simulink library "halout"  (R2021b)
settings: Solver=VariableStepAuto  StartTime=0.0  StopTime=10.0  RelTol=1e-3
undefined symbols (not defined in the file): C_TASK_5MS_S, KHAL_CAN1TxReq_flg, KHAL_CAN2TxReq_flg, KHAL_CAN3TxReq_flg, KHAL_CAN4TxReq_flg, KHAL_CAN5TxReq_flg, KHAL_CAN6TxReq_flg, KHAL_CAN7TxReq_flg, TRUE
libraries: FVT_lib x65, simulink x6
(part 5 of 6)

== system halout/HAL_OUT/CAN2/FD2_CE100_0_0x209/FDCBCMBSDBuzzerCmd ==
  FDCBCMBSDBuzzerCmd : Inport
  Data Type Conversion : DataTypeConversion  OutDataTypeStr=uint8  RndMeth=Round
  CAN2_FDC_BCM_BSD_Buzzer_Cmd : Outport
  wires:
  Data Type Conversion/1 -> CAN2_FDC_BCM_BSD_Buzzer_Cmd/1
  FDCBCMBSDBuzzerCmd/1 -> Data Type Conversion/1

== system halout/HAL_OUT/CAN2/FD2_CE100_0_0x209/FDCBCMBrakeCmd ==
  FDCBCMBrakeCmd : Inport
  Data Type Conversion : DataTypeConversion  OutDataTypeStr=uint8  RndMeth=Round
  CAN2_FDC_BCM_Brake_Cmd : Outport
  wires:
  Data Type Conversion/1 -> CAN2_FDC_BCM_Brake_Cmd/1
  FDCBCMBrakeCmd/1 -> Data Type Conversion/1

== system halout/HAL_OUT/CAN2/FD2_CE100_0_0x209/FDCBCMCallBellCmd ==
  FDCBCMCallBellCmd : Inport
  Data Type Conversion : DataTypeConversion  OutDataTypeStr=uint8  RndMeth=Round
  CAN2_FDC_BCM_CallBell_Cmd : Outport
  wires:
  Data Type Conversion/1 -> CAN2_FDC_BCM_CallBell_Cmd/1
  FDCBCMCallBellCmd/1 -> Data Type Conversion/1

== system halout/HAL_OUT/CAN2/FD2_CE100_0_0x209/FDCBCMDVRSignalLCmd ==
  FDCBCMDVRSignalLCmd : Inport
  Data Type Conversion : DataTypeConversion  OutDataTypeStr=uint8  RndMeth=Round
  CAN2_FDC_BCM_DVRSignalL_Cmd : Outport
  wires:
  Data Type Conversion/1 -> CAN2_FDC_BCM_DVRSignalL_Cmd/1
  FDCBCMDVRSignalLCmd/1 -> Data Type Conversion/1

== system halout/HAL_OUT/CAN2/FD2_CE100_0_0x209/FDCBCMDVRSignalRCmd ==
  FDCBCMDVRSignalRCmd : Inport
  Data Type Conversion : DataTypeConversion  OutDataTypeStr=uint8  RndMeth=Round
  CAN2_FDC_BCM_DVRSignalR_Cmd : Outport
  wires:
  Data Type Conversion/1 -> CAN2_FDC_BCM_DVRSignalR_Cmd/1
  FDCBCMDVRSignalRCmd/1 -> Data Type Conversion/1

== system halout/HAL_OUT/CAN2/FD2_CE100_0_0x209/FDCBCMEmExitSWSta ==
  FDCBCMEmExitSWSta : Inport
  Data Type Conversion : DataTypeConversion  OutDataTypeStr=uint8  RndMeth=Round
  CAN2_FDC_BCM_EmExitSW_Sta : Outport
  wires:
  Data Type Conversion/1 -> CAN2_FDC_BCM_EmExitSW_Sta/1
  FDCBCMEmExitSWSta/1 -> Data Type Conversion/1

== system halout/HAL_OUT/CAN2/FD2_CE100_0_0x209/FDCBCMEmSVCmd ==
  FDCBCMEmSVCmd : Inport
  Data Type Conversion : DataTypeConversion  OutDataTypeStr=uint8  RndMeth=Round
  CAN2_FDC_BCM_EmSV_Cmd : Outport
  wires:
  Data Type Conversion/1 -> CAN2_FDC_BCM_EmSV_Cmd/1
  FDCBCMEmSVCmd/1 -> Data Type Conversion/1

== system halout/HAL_OUT/CAN2/FD2_CE100_0_0x209/FDCBCMFDCloseSVCmd ==
  FDCBCMFDCloseSVCmd : Inport
  Data Type Conversion : DataTypeConversion  OutDataTypeStr=uint8  RndMeth=Round
  CAN2_FDC_BCM_FDCloseSV_Cmd : Outport
  wires:
  Data Type Conversion/1 -> CAN2_FDC_BCM_FDCloseSV_Cmd/1
  FDCBCMFDCloseSVCmd/1 -> Data Type Conversion/1

== system halout/HAL_OUT/CAN2/FD2_CE100_0_0x209/FDCBCMFDOpenSVCmd ==
  FDCBCMFDOpenSVCmd : Inport
  Data Type Conversion : DataTypeConversion  OutDataTypeStr=uint8  RndMeth=Round
  CAN2_FDC_BCM_FDOpenSV_Cmd : Outport
  wires:
  Data Type Conversion/1 -> CAN2_FDC_BCM_FDOpenSV_Cmd/1
  FDCBCMFDOpenSVCmd/1 -> Data Type Conversion/1

== system halout/HAL_OUT/CAN2/FD2_CE100_0_0x209/FDCBCMFDoorSta ==
  FDCBCMFDoorSta : Inport
  Data Type Conversion : DataTypeConversion  OutDataTypeStr=uint8  RndMeth=Round
  CAN2_FDC_BCM_FDoor_Sta : Outport
  wires:
  Data Type Conversion/1 -> CAN2_FDC_BCM_FDoor_Sta/1
  FDCBCMFDoorSta/1 -> Data Type Conversion/1

== system halout/HAL_OUT/CAN2/FD2_CE100_0_0x209/FDCBCMFRoomLpSetSta ==
  FDCBCMFRoomLpSetSta : Inport
  Data Type Conversion : DataTypeConversion  OutDataTypeStr=uint8  RndMeth=Round
  CAN2_FDC_BCM_FRoomLpSet_Sta : Outport
  wires:
  Data Type Conversion/1 -> CAN2_FDC_BCM_FRoomLpSet_Sta/1
  FDCBCMFRoomLpSetSta/1 -> Data Type Conversion/1

== system halout/HAL_OUT/CAN2/FD2_CE100_0_0x209/FDCBCMHBeamCmd ==
  FDCBCMHBeamCmd : Inport
  Data Type Conversion : DataTypeConversion  OutDataTypeStr=uint8  RndMeth=Round
  CAN2_FDC_BCM_HBeam_Cmd : Outport
  wires:
  Data Type Conversion/1 -> CAN2_FDC_BCM_HBeam_Cmd/1
  FDCBCMHBeamCmd/1 -> Data Type Conversion/1

== system halout/HAL_OUT/CAN2/FD2_CE100_0_0x209/FDCBCMHazardSWSta ==
  FDCBCMHazardSWSta : Inport
  Data Type Conversion : DataTypeConversion  OutDataTypeStr=uint8  RndMeth=Round
  CAN2_FDC_BCM_HazardSW_Sta : Outport
  wires:
  Data Type Conversion/1 -> CAN2_FDC_BCM_HazardSW_Sta/1
  FDCBCMHazardSWSta/1 -> Data Type Conversion/1

== system halout/HAL_OUT/CAN2/FD2_CE100_0_0x209/FDCBCMHelpINDCmd ==
  FDCBCMHelpINDCmd : Inport
  Data Type Conversion : DataTypeConversion  OutDataTypeStr=uint8  RndMeth=Round
  CAN2_FDC_BCM_HelpIND_Cmd : Outport
  wires:
  Data Type Conversion/1 -> CAN2_FDC_BCM_HelpIND_Cmd/1
  FDCBCMHelpINDCmd/1 -> Data Type Conversion/1

== system halout/HAL_OUT/CAN2/FD2_CE100_0_0x209/FDCBCMInnerBuzzerCmd ==
  FDCBCMInnerBuzzerCmd : Inport
  Data Type Conversion : DataTypeConversion  OutDataTypeStr=uint8  RndMeth=Round
  CAN2_FDC_BCM_InnerBuzzer_Cmd : Outport
  wires:
  Data Type Conversion/1 -> CAN2_FDC_BCM_InnerBuzzer_Cmd/1
  FDCBCMInnerBuzzerCmd/1 -> Data Type Conversion/1

== system halout/HAL_OUT/CAN2/FD2_CE100_0_0x209/FDCBCMInnerBuzzerModeSta ==
  FDCBCMInnerBuzzerModeSta : Inport
  Data Type Conversion : DataTypeConversion  OutDataTypeStr=uint8  RndMeth=Round
  CAN2_FDC_BCM_InnerBuzzerMode_Sta : Outport
  wires:
  Data Type Conversion/1 -> CAN2_FDC_BCM_InnerBuzzerMode_Sta/1
  FDCBCMInnerBuzzerModeSta/1 -> Data Type Conversion/1

== system halout/HAL_OUT/CAN2/FD2_CE100_0_0x209/FDCBCMInnerCallBellCmd ==
  FDCBCMInnerCallBellCmd : Inport
  Data Type Conversion : DataTypeConversion  OutDataTypeStr=uint8  RndMeth=Round
  CAN2_FDC_BCM_InnerCallBell_Cmd : Outport
  wires:
  Data Type Conversion/1 -> CAN2_FDC_BCM_InnerCallBell_Cmd/1
  FDCBCMInnerCallBellCmd/1 -> Data Type Conversion/1

== system halout/HAL_OUT/CAN2/FD2_CE100_0_0x209/FDCBCMLBSDRCmd ==
  FDCBCMLBSDRCmd : Inport
  Data Type Conversion : DataTypeConversion  OutDataTypeStr=uint8  RndMeth=Round
  CAN2_FDC_BCM_LBSDR_Cmd : Outport
  wires:
  Data Type Conversion/1 -> CAN2_FDC_BCM_LBSDR_Cmd/1
  FDCBCMLBSDRCmd/1 -> Data Type Conversion/1

== system halout/HAL_OUT/CAN2/FD2_CE100_0_0x209/FDCBCMLBSDYCmd ==
  FDCBCMLBSDYCmd : Inport
  Data Type Conversion : DataTypeConversion  OutDataTypeStr=uint8  RndMeth=Round
  CAN2_FDC_BCM_LBSDY_Cmd : Outport
  wires:
  Data Type Conversion/1 -> CAN2_FDC_BCM_LBSDY_Cmd/1
  FDCBCMLBSDYCmd/1 -> Data Type Conversion/1

== system halout/HAL_OUT/CAN2/FD2_CE100_0_0x209/FDCBCMLBeamCmd ==
  FDCBCMLBeamCmd : Inport
  Data Type Conversion : DataTypeConversion  OutDataTypeStr=uint8  RndMeth=Round
  CAN2_FDC_BCM_LBeam_Cmd : Outport
  wires:
  Data Type Conversion/1 -> CAN2_FDC_BCM_LBeam_Cmd/1
  FDCBCMLBeamCmd/1 -> Data Type Conversion/1

== system halout/HAL_OUT/CAN2/FD2_CE100_0_0x209/FDCBCMLDRLCmd ==
  FDCBCMLDRLCmd : Inport
  Data Type Conversion : DataTypeConversion  OutDataTypeStr=uint8  RndMeth=Round
  CAN2_FDC_BCM_LDRL_Cmd : Outport
  wires:
  Data Type Conversion/1 -> CAN2_FDC_BCM_LDRL_Cmd/1
  FDCBCMLDRLCmd/1 -> Data Type Conversion/1

== system halout/HAL_OUT/CAN2/FD2_CE100_0_0x209/FDCBCMLTurnLpCmd ==
  FDCBCMLTurnLpCmd : Inport
  Data Type Conversion : DataTypeConversion  OutDataTypeStr=uint8  RndMeth=Round
  CAN2_FDC_BCM_LTurnLp_Cmd : Outport
  wires:
  Data Type Conversion/1 -> CAN2_FDC_BCM_LTurnLp_Cmd/1
  FDCBCMLTurnLpCmd/1 -> Data Type Conversion/1

== system halout/HAL_OUT/CAN2/FD2_CE100_0_0x209/FDCBCMLTurnSWSta ==
  FDCBCMLTurnSWSta : Inport
  Data Type Conversion : DataTypeConversion  OutDataTypeStr=uint8  RndMeth=Round
  CAN2_FDC_BCM_LTurnSW_Sta : Outport
  wires:
  Data Type Conversion/1 -> CAN2_FDC_BCM_LTurnSW_Sta/1
  FDCBCMLTurnSWSta/1 -> Data Type Conversion/1

== system halout/HAL_OUT/CAN2/FD2_CE100_0_0x209/FDCBCMMDCloseSVCmd ==
  FDCBCMMDCloseSVCmd : Inport
  Data Type Conversion : DataTypeConversion  OutDataTypeStr=uint8  RndMeth=Round
  CAN2_FDC_BCM_MDCloseSV_Cmd : Outport
  wires:
  Data Type Conversion/1 -> CAN2_FDC_BCM_MDCloseSV_Cmd/1
  FDCBCMMDCloseSVCmd/1 -> Data Type Conversion/1

== system halout/HAL_OUT/CAN2/FD2_CE100_0_0x209/FDCBCMMDOpenSVCmd ==
  FDCBCMMDOpenSVCmd : Inport
  Data Type Conversion : DataTypeConversion  OutDataTypeStr=uint8  RndMeth=Round
  CAN2_FDC_BCM_MDOpenSV_Cmd : Outport
  wires:
  Data Type Conversion/1 -> CAN2_FDC_BCM_MDOpenSV_Cmd/1
  FDCBCMMDOpenSVCmd/1 -> Data Type Conversion/1

== system halout/HAL_OUT/CAN2/FD2_CE100_0_0x209/FDCBCMMDoorSta ==
  FDCBCMMDoorSta : Inport
  Data Type Conversion : DataTypeConversion  OutDataTypeStr=uint8  RndMeth=Round
  CAN2_FDC_BCM_MDoor_Sta : Outport
  wires:
  Data Type Conversion/1 -> CAN2_FDC_BCM_MDoor_Sta/1
  FDCBCMMDoorSta/1 -> Data Type Conversion/1

== system halout/HAL_OUT/CAN2/FD2_CE100_0_0x209/FDCBCMMRoomLpSetSta ==
  FDCBCMMRoomLpSetSta : Inport
  Data Type Conversion : DataTypeConversion  OutDataTypeStr=uint8  RndMeth=Round
  CAN2_FDC_BCM_MRoomLpSet_Sta : Outport
  wires:
  Data Type Conversion/1 -> CAN2_FDC_BCM_MRoomLpSet_Sta/1
  FDCBCMMRoomLpSetSta/1 -> Data Type Conversion/1

== system halout/HAL_OUT/CAN2/FD2_CE100_0_0x209/FDCBCMOutDoorOpenSWSta ==
  FDCBCMOutDoorOpenSWSta : Inport
  Data Type Conversion : DataTypeConversion  OutDataTypeStr=uint8  RndMeth=Round
  CAN2_FDC_BCM_OutDoorOpenSW_Sta : Outport
  wires:
  Data Type Conversion/1 -> CAN2_FDC_BCM_OutDoorOpenSW_Sta/1
  FDCBCMOutDoorOpenSWSta/1 -> Data Type Conversion/1

== system halout/HAL_OUT/CAN2/FD2_CE100_0_0x209/FDCBCMPLampCmd ==
  FDCBCMPLampCmd : Inport
  Data Type Conversion : DataTypeConversion  OutDataTypeStr=uint8  RndMeth=Round
  CAN2_FDC_BCM_PLamp_Cmd : Outport
  wires:
  Data Type Conversion/1 -> CAN2_FDC_BCM_PLamp_Cmd/1
  FDCBCMPLampCmd/1 -> Data Type Conversion/1

== system halout/HAL_OUT/CAN2/FD2_CE100_0_0x209/FDCBCMRBSDRCmd ==
  FDCBCMRBSDRCmd : Inport
  Data Type Conversion : DataTypeConversion  OutDataTypeStr=uint8  RndMeth=Round
  CAN2_FDC_BCM_RBSDR_Cmd : Outport
  wires:
  Data Type Conversion/1 -> CAN2_FDC_BCM_RBSDR_Cmd/1
  FDCBCMRBSDRCmd/1 -> Data Type Conversion/1

== system halout/HAL_OUT/CAN2/FD2_CE100_0_0x209/FDCBCMRBSDYCmd ==
  FDCBCMRBSDYCmd : Inport
  Data Type Conversion : DataTypeConversion  OutDataTypeStr=uint8  RndMeth=Round
  CAN2_FDC_BCM_RBSDY_Cmd : Outport
  wires:
  Data Type Conversion/1 -> CAN2_FDC_BCM_RBSDY_Cmd/1
  FDCBCMRBSDYCmd/1 -> Data Type Conversion/1

== system halout/HAL_OUT/CAN2/FD2_CE100_0_0x209/FDCBCMRDRLCmd ==
  FDCBCMRDRLCmd : Inport
  Data Type Conversion : DataTypeConversion  OutDataTypeStr=uint8  RndMeth=Round
  CAN2_FDC_BCM_RDRL_Cmd : Outport
  wires:
  Data Type Conversion/1 -> CAN2_FDC_BCM_RDRL_Cmd/1
  FDCBCMRDRLCmd/1 -> Data Type Conversion/1

== system halout/HAL_OUT/CAN2/FD2_CE100_0_0x209/FDCBCMRDoorSta ==
  FDCBCMRDoorSta : Inport
  Data Type Conversion : DataTypeConversion  OutDataTypeStr=uint8  RndMeth=Round
  CAN2_FDC_BCM_RDoor_Sta : Outport
  wires:
  Data Type Conversion/1 -> CAN2_FDC_BCM_RDoor_Sta/1
  FDCBCMRDoorSta/1 -> Data Type Conversion/1

== system halout/HAL_OUT/CAN2/FD2_CE100_0_0x209/FDCBCMRFLampCmd ==
  FDCBCMRFLampCmd : Inport
  Data Type Conversion : DataTypeConversion  OutDataTypeStr=uint8  RndMeth=Round
  CAN2_FDC_BCM_RFLamp_Cmd : Outport
  wires:
  Data Type Conversion/1 -> CAN2_FDC_BCM_RFLamp_Cmd/1
  FDCBCMRFLampCmd/1 -> Data Type Conversion/1

== system halout/HAL_OUT/CAN2/FD2_CE100_0_0x209/FDCBCMRGearSta ==
  FDCBCMRGearSta : Inport
  Data Type Conversion : DataTypeConversion  OutDataTypeStr=uint8  RndMeth=Round
  CAN2_FDC_BCM_RGear_Sta : Outport
  wires:
  Data Type Conversion/1 -> CAN2_FDC_BCM_RGear_Sta/1
  FDCBCMRGearSta/1 -> Data Type Conversion/1

== system halout/HAL_OUT/CAN2/FD2_CE100_0_0x209/FDCBCMRRoomLpSetSta ==
  FDCBCMRRoomLpSetSta : Inport
  Data Type Conversion : DataTypeConversion  OutDataTypeStr=uint8  RndMeth=Round
  CAN2_FDC_BCM_RRoomLpSet_Sta : Outport
  wires:
  Data Type Conversion/1 -> CAN2_FDC_BCM_RRoomLpSet_Sta/1
  FDCBCMRRoomLpSetSta/1 -> Data Type Conversion/1

== system halout/HAL_OUT/CAN2/FD2_CE100_0_0x209/FDCBCMRTurnLpCmd ==
  FDCBCMRTurnLpCmd : Inport
  Data Type Conversion : DataTypeConversion  OutDataTypeStr=uint8  RndMeth=Round
  CAN2_FDC_BCM_RTurnLp_Cmd : Outport
  wires:
  Data Type Conversion/1 -> CAN2_FDC_BCM_RTurnLp_Cmd/1
  FDCBCMRTurnLpCmd/1 -> Data Type Conversion/1

== system halout/HAL_OUT/CAN2/FD2_CE100_0_0x209/FDCBCMRTurnSWSta ==
  FDCBCMRTurnSWSta : Inport
  Data Type Conversion : DataTypeConversion  OutDataTypeStr=uint8  RndMeth=Round
  CAN2_FDC_BCM_RTurnSW_Sta : Outport
  wires:
  Data Type Conversion/1 -> CAN2_FDC_BCM_RTurnSW_Sta/1
  FDCBCMRTurnSWSta/1 -> Data Type Conversion/1

== system halout/HAL_OUT/CAN2/FD2_CE100_0_0x209/FDCBCMRoomLpAmbCmd ==
  FDCBCMRoomLpAmbCmd : Inport
  Data Type Conversion : DataTypeConversion  OutDataTypeStr=uint8  RndMeth=Round
  CAN2_FDC_BCM_RoomLpAmb_Cmd : Outport
  wires:
  Data Type Conversion/1 -> CAN2_FDC_BCM_RoomLpAmb_Cmd/1
  FDCBCMRoomLpAmbCmd/1 -> Data Type Conversion/1

== system halout/HAL_OUT/CAN2/FD2_CE100_0_0x209/FDCBCMRoomLpAmbSetSta ==
  FDCBCMRoomLpAmbSetSta : Inport
  Data Type Conversion : DataTypeConversion  OutDataTypeStr=uint8  RndMeth=Round
  CAN2_FDC_BCM_RoomLpAmbSet_Sta : Outport
  wires:
  Data Type Conversion/1 -> CAN2_FDC_BCM_RoomLpAmbSet_Sta/1
  FDCBCMRoomLpAmbSetSta/1 -> Data Type Conversion/1

== system halout/HAL_OUT/CAN2/FD2_CE100_0_0x209/FDCBCMRoomLpSetSta ==
  FDCBCMRoomLpSetSta : Inport
  Data Type Conversion : DataTypeConversion  OutDataTypeStr=uint8  RndMeth=Round
  CAN2_FDC_BCM_RoomLpSet_Sta : Outport
  wires:
  Data Type Conversion/1 -> CAN2_FDC_BCM_RoomLpSet_Sta/1
  FDCBCMRoomLpSetSta/1 -> Data Type Conversion/1

== system halout/HAL_OUT/CAN2/FD2_CE100_0_0x209/FDCBCMSLTLpCmd ==
  FDCBCMSLTLpCmd : Inport
  Data Type Conversion : DataTypeConversion  OutDataTypeStr=uint8  RndMeth=Round
  CAN2_FDC_BCM_SLTLp_Cmd : Outport
  wires:
  Data Type Conversion/1 -> CAN2_FDC_BCM_SLTLp_Cmd/1
  FDCBCMSLTLpCmd/1 -> Data Type Conversion/1

== system halout/HAL_OUT/CAN2/FD2_CE100_0_0x209/FDCBCMSMKLCmd ==
  FDCBCMSMKLCmd : Inport
  Data Type Conversion : DataTypeConversion  OutDataTypeStr=uint8  RndMeth=Round
  CAN2_FDC_BCM_SMKL_Cmd : Outport
  wires:
  Data Type Conversion/1 -> CAN2_FDC_BCM_SMKL_Cmd/1
  FDCBCMSMKLCmd/1 -> Data Type Conversion/1

== system halout/HAL_OUT/CAN2/FD2_CE100_0_0x209/FDCBCMSMKRCmd ==
  FDCBCMSMKRCmd : Inport
  Data Type Conversion : DataTypeConversion  OutDataTypeStr=uint8  RndMeth=Round
  CAN2_FDC_BCM_SMKR_Cmd : Outport
  wires:
  Data Type Conversion/1 -> CAN2_FDC_BCM_SMKR_Cmd/1
  FDCBCMSMKRCmd/1 -> Data Type Conversion/1

== system halout/HAL_OUT/CAN2/FD2_CE100_0_0x209/FDCBCMSRTLpCmd ==
  FDCBCMSRTLpCmd : Inport
  Data Type Conversion : DataTypeConversion  OutDataTypeStr=uint8  RndMeth=Round
  CAN2_FDC_BCM_SRTLp_Cmd : Outport
  wires:
  Data Type Conversion/1 -> CAN2_FDC_BCM_SRTLp_Cmd/1
  FDCBCMSRTLpCmd/1 -> Data Type Conversion/1

== system halout/HAL_OUT/CAN2/FD2_CE100_0_0x209/FDCBCMSTOPBALLCmd ==
  FDCBCMSTOPBALLCmd : Inport
  Data Type Conversion : DataTypeConversion  OutDataTypeStr=uint8  RndMeth=Round
  CAN2_FDC_BCM_STOPBALL_Cmd : Outport
  wires:
  Data Type Conversion/1 -> CAN2_FDC_BCM_STOPBALL_Cmd/1
  FDCBCMSTOPBALLCmd/1 -> Data Type Conversion/1

== system halout/HAL_OUT/CAN2/FD2_CE100_0_0x209/FDCBCMStopINDCmd ==
  FDCBCMStopINDCmd : Inport
  Data Type Conversion : DataTypeConversion  OutDataTypeStr=uint8  RndMeth=Round
  CAN2_FDC_BCM_Stop_IND_Cmd : Outport
  wires:
  Data Type Conversion/1 -> CAN2_FDC_BCM_Stop_IND_Cmd/1
  FDCBCMStopINDCmd/1 -> Data Type Conversion/1

== system halout/HAL_OUT/CAN2/FD2_CE100_0_0x209/FDCBCMTurnBuzzerENSta ==
  FDCBCMTurnBuzzerENSta : Inport
  Data Type Conversion : DataTypeConversion  OutDataTypeStr=uint8  RndMeth=Round
  CAN2_FDC_BCM_TurnBuzzerEN_Sta : Outport
  wires:
  Data Type Conversion/1 -> CAN2_FDC_BCM_TurnBuzzerEN_Sta/1
  FDCBCMTurnBuzzerENSta/1 -> Data Type Conversion/1

== system halout/HAL_OUT/CAN2/FD2_CE100_0_0x209/FDCBCMTurnLpPatternSta ==
  FDCBCMTurnLpPatternSta : Inport
  Data Type Conversion : DataTypeConversion  OutDataTypeStr=uint8  RndMeth=Round
  CAN2_FDC_BCM_TurnLpPattern_Sta : Outport
  wires:
  Data Type Conversion/1 -> CAN2_FDC_BCM_TurnLpPattern_Sta/1
  FDCBCMTurnLpPatternSta/1 -> Data Type Conversion/1

== system halout/HAL_OUT/CAN2/FD2_CE100_0_0x209/FDCBCMWasherCmd ==
  FDCBCMWasherCmd : Inport
  Data Type Conversion : DataTypeConversion  OutDataTypeStr=uint8  RndMeth=Round
  CAN2_FDC_BCM_Washer_Cmd : Outport
  wires:
  Data Type Conversion/1 -> CAN2_FDC_BCM_Washer_Cmd/1
  FDCBCMWasherCmd/1 -> Data Type Conversion/1

== system halout/HAL_OUT/CAN2/FD2_CE100_0_0x209/FDCBCMWiperHCmd ==
  FDCBCMWiperHCmd : Inport
  Data Type Conversion : DataTypeConversion  OutDataTypeStr=uint8  RndMeth=Round
  CAN2_FDC_BCM_WiperH_Cmd : Outport
  wires:
  Data Type Conversion/1 -> CAN2_FDC_BCM_WiperH_Cmd/1
  FDCBCMWiperHCmd/1 -> Data Type Conversion/1

== system halout/HAL_OUT/CAN2/FD2_CE100_0_0x209/FDCBCMWiperLCmd ==
  FDCBCMWiperLCmd : Inport
  Data Type Conversion : DataTypeConversion  OutDataTypeStr=uint8  RndMeth=Round
  CAN2_FDC_BCM_WiperL_Cmd : Outport
  wires:
  Data Type Conversion/1 -> CAN2_FDC_BCM_WiperL_Cmd/1
  FDCBCMWiperLCmd/1 -> Data Type Conversion/1

== system halout/HAL_OUT/CAN2/GW2_C100_0_0x20B/CACTempWarn ==
  CACTempWarn : Inport
  Data Type Conversion : DataTypeConversion  OutDataTypeStr=uint8  RndMeth=Round
  CAN2_CACTempWarn : Outport
  wires:
  Data Type Conversion/1 -> CAN2_CACTempWarn/1
  CACTempWarn/1 -> Data Type Conversion/1

== system halout/HAL_OUT/CAN2/GW2_C100_0_0x20B/DACStatus ==
  DACStatus : Inport
  Data Type Conversion : DataTypeConversion  OutDataTypeStr=uint8  RndMeth=Round
  CAN2_DACStatus : Outport
  wires:
  Data Type Conversion/1 -> CAN2_DACStatus/1
  DACStatus/1 -> Data Type Conversion/1

== system halout/HAL_OUT/CAN2/GW2_C100_0_0x20B/GearFlashInd ==
  GearFlashInd : Inport
  Data Type Conversion : DataTypeConversion  OutDataTypeStr=uint8  RndMeth=Round
  CAN2_GearFlashInd : Outport
  wires:
  Data Type Conversion/1 -> CAN2_GearFlashInd/1
  GearFlashInd/1 -> Data Type Conversion/1

== system halout/HAL_OUT/CAN2/GW2_C100_0_0x20B/LVBattLow ==
  LVBattLow : Inport
  Data Type Conversion : DataTypeConversion  OutDataTypeStr=uint8  RndMeth=Round
  CAN2_LVBattLow : Outport
  wires:
  Data Type Conversion/1 -> CAN2_LVBattLow/1
  LVBattLow/1 -> Data Type Conversion/1

== system halout/HAL_OUT/CAN2/GW2_C100_0_0x20B/PweLmtInd ==
  PweLmtInd : Inport
  Data Type Conversion : DataTypeConversion  OutDataTypeStr=uint8  RndMeth=Round
  CAN2_PweLmtInd : Outport
  wires:
  Data Type Conversion/1 -> CAN2_PweLmtInd/1
  PweLmtInd/1 -> Data Type Conversion/1

== system halout/HAL_OUT/CAN2/GW2_C100_0_0x20B/VCUWarnInd ==
  VCUWarnInd : Inport
  Data Type Conversion : DataTypeConversion  OutDataTypeStr=uint8  RndMeth=Round
  CAN2_VCUWarnInd : Outport
  wires:
  Data Type Conversion/1 -> CAN2_VCUWarnInd/1
  VCUWarnInd/1 -> Data Type Conversion/1

== system halout/HAL_OUT/CAN2/GW2_C100_0_0x20B/VCUnoPBInd ==
  VCUnoPBInd : Inport
  Data Type Conversion : DataTypeConversion  OutDataTypeStr=uint8  RndMeth=Round
  CAN2_VCUnoPBInd : Outport
  wires:
  Data Type Conversion/1 -> CAN2_VCUnoPBInd/1
  VCUnoPBInd/1 -> Data Type Conversion/1

== system halout/HAL_OUT/CAN3/FD3_C100_0_0x1802F3EF/V2BACPosRlyFlt ==
  V2BACPosRlyFlt : Inport
  Data Type Conversion : DataTypeConversion  OutDataTypeStr=uint8  RndMeth=Round
  CAN3_V2BACPosRlyFlt : Outport
  wires:
  Data Type Conversion/1 -> CAN3_V2BACPosRlyFlt/1
  V2BACPosRlyFlt/1 -> Data Type Conversion/1

== system halout/HAL_OUT/CAN3/FD3_C100_0_0x1802F3EF/V2BACPosRlySta ==
  V2BACPosRlySta : Inport
  Data Type Conversion : DataTypeConversion  OutDataTypeStr=uint8  RndMeth=Round
  CAN3_V2BACPosRlySta : Outport
  wires:
  Data Type Conversion/1 -> CAN3_V2BACPosRlySta/1
  V2BACPosRlySta/1 -> Data Type Conversion/1

== system halout/HAL_OUT/CAN3/FD3_C100_0_0x1802F3EF/V2BAirPosRlyFlt ==
  V2BAirPosRlyFlt : Inport
  Data Type Conversion : DataTypeConversion  OutDataTypeStr=uint8  RndMeth=Round
  CAN3_V2BAirPosRlyFlt : Outport
  wires:
  Data Type Conversion/1 -> CAN3_V2BAirPosRlyFlt/1
  V2BAirPosRlyFlt/1 -> Data Type Conversion/1

== system halout/HAL_OUT/CAN3/FD3_C100_0_0x1802F3EF/V2BAirPosRlySta ==
  V2BAirPosRlySta : Inport
  Data Type Conversion : DataTypeConversion  OutDataTypeStr=uint8  RndMeth=Round
  CAN3_V2BAirPosRlySta : Outport
  wires:
  Data Type Conversion/1 -> CAN3_V2BAirPosRlySta/1
  V2BAirPosRlySta/1 -> Data Type Conversion/1

== system halout/HAL_OUT/CAN3/FD3_C100_0_0x1802F3EF/V2BAux1OnOff ==
  V2BAux1OnOff : Inport
  Data Type Conversion : DataTypeConversion  OutDataTypeStr=uint8  RndMeth=Round
  CAN3_V2BAux1OnOff : Outport
  wires:
  Data Type Conversion/1 -> CAN3_V2BAux1OnOff/1
  V2BAux1OnOff/1 -> Data Type Conversion/1

== system halout/HAL_OUT/CAN3/FD3_C100_0_0x1802F3EF/V2BAux1RlyFlt ==
  V2BAux1RlyFlt : Inport
  Data Type Conversion : DataTypeConversion  OutDataTypeStr=uint8  RndMeth=Round
  CAN3_V2BAux1RlyFlt : Outport
  wires:
  Data Type Conversion/1 -> CAN3_V2BAux1RlyFlt/1
  V2BAux1RlyFlt/1 -> Data Type Conversion/1

== system halout/HAL_OUT/CAN3/FD3_C100_0_0x1802F3EF/V2BAux1RlySta ==
  V2BAux1RlySta : Inport
  Data Type Conversion : DataTypeConversion  OutDataTypeStr=uint8  RndMeth=Round
  CAN3_V2BAux1RlySta : Outport
  wires:
  Data Type Conversion/1 -> CAN3_V2BAux1RlySta/1
  V2BAux1RlySta/1 -> Data Type Conversion/1

== system halout/HAL_OUT/CAN3/FD3_C100_0_0x1802F3EF/V2BAux2OnOff ==
  V2BAux2OnOff : Inport
  Data Type Conversion : DataTypeConversion  OutDataTypeStr=uint8  RndMeth=Round
  CAN3_V2BAux2OnOff : Outport
  wires:
  Data Type Conversion/1 -> CAN3_V2BAux2OnOff/1
  V2BAux2OnOff/1 -> Data Type Conversion/1

== system halout/HAL_OUT/CAN3/FD3_C100_0_0x1802F3EF/V2BAux2RlyFlt ==
  V2BAux2RlyFlt : Inport
  Data Type Conversion : DataTypeConversion  OutDataTypeStr=uint8  RndMeth=Round
  CAN3_V2BAux2RlyFlt : Outport
  wires:
  Data Type Conversion/1 -> CAN3_V2BAux2RlyFlt/1
  V2BAux2RlyFlt/1 -> Data Type Conversion/1

== system halout/HAL_OUT/CAN3/FD3_C100_0_0x1802F3EF/V2BAux2RlySta ==
  V2BAux2RlySta : Inport
  Data Type Conversion : DataTypeConversion  OutDataTypeStr=uint8  RndMeth=Round
  CAN3_V2BAux2RlySta : Outport
  wires:
  Data Type Conversion/1 -> CAN3_V2BAux2RlySta/1
  V2BAux2RlySta/1 -> Data Type Conversion/1

== system halout/HAL_OUT/CAN3/FD3_C100_0_0x1802F3EF/V2BAux3OnOff ==
  V2BAux3OnOff : Inport
  Data Type Conversion : DataTypeConversion  OutDataTypeStr=uint8  RndMeth=Round
  CAN3_V2BAux3OnOff : Outport
  wires:
  Data Type Conversion/1 -> CAN3_V2BAux3OnOff/1
  V2BAux3OnOff/1 -> Data Type Conversion/1

== system halout/HAL_OUT/CAN3/FD3_C100_0_0x1802F3EF/V2BAux3RlyFlt ==
  V2BAux3RlyFlt : Inport
  Data Type Conversion : DataTypeConversion  OutDataTypeStr=uint8  RndMeth=Round
  CAN3_V2BAux3RlyFlt : Outport
  wires:
  Data Type Conversion/1 -> CAN3_V2BAux3RlyFlt/1
  V2BAux3RlyFlt/1 -> Data Type Conversion/1

== system halout/HAL_OUT/CAN3/FD3_C100_0_0x1802F3EF/V2BAux3RlySta ==
  V2BAux3RlySta : Inport
  Data Type Conversion : DataTypeConversion  OutDataTypeStr=uint8  RndMeth=Round
  CAN3_V2BAux3RlySta : Outport
  wires:
  Data Type Conversion/1 -> CAN3_V2BAux3RlySta/1
  V2BAux3RlySta/1 -> Data Type Conversion/1

== system halout/HAL_OUT/CAN3/FD3_C100_0_0x1802F3EF/V2BAux4ReyFlt ==
  V2BAux4ReyFlt : Inport
  Data Type Conversion : DataTypeConversion  OutDataTypeStr=uint8  RndMeth=Round
  CAN3_V2BAux4ReyFlt : Outport
  wires:
  Data Type Conversion/1 -> CAN3_V2BAux4ReyFlt/1
  V2BAux4ReyFlt/1 -> Data Type Conversion/1

== system halout/HAL_OUT/CAN3/FD3_C100_0_0x1802F3EF/V2BAux4RlySta ==
  V2BAux4RlySta : Inport
  Data Type Conversion : DataTypeConversion  OutDataTypeStr=uint8  RndMeth=Round
  CAN3_V2BAux4RlySta : Outport
  wires:
  Data Type Conversion/1 -> CAN3_V2BAux4RlySta/1
  V2BAux4RlySta/1 -> Data Type Conversion/1

== system halout/HAL_OUT/CAN3/FD3_C100_0_0x1802F3EF/V2BDCDCPosRlyFlt ==
  V2BDCDCPosRlyFlt : Inport
  Data Type Conversion : DataTypeConversion  OutDataTypeStr=uint8  RndMeth=Round
  CAN3_V2BDCDCPosRlyFlt : Outport
  wires:
  Data Type Conversion/1 -> CAN3_V2BDCDCPosRlyFlt/1
  V2BDCDCPosRlyFlt/1 -> Data Type Conversion/1

== system halout/HAL_OUT/CAN3/FD3_C100_0_0x1802F3EF/V2BDCDCPosRlySta ==
  V2BDCDCPosRlySta : Inport
  Data Type Conversion : DataTypeConversion  OutDataTypeStr=uint8  RndMeth=Round
  CAN3_V2BDCDCPosRlySta : Outport
  wires:
  Data Type Conversion/1 -> CAN3_V2BDCDCPosRlySta/1
  V2BDCDCPosRlySta/1 -> Data Type Conversion/1

== system halout/HAL_OUT/CAN3/FD3_C100_0_0x1802F3EF/V2BHVOnOff ==
  V2BHVOnOff : Inport
  Data Type Conversion : DataTypeConversion  OutDataTypeStr=uint8  RndMeth=Round
  CAN3_V2BHVOnOff : Outport
  wires:
  Data Type Conversion/1 -> CAN3_V2BHVOnOff/1
  V2BHVOnOff/1 -> Data Type Conversion/1

== system halout/HAL_OUT/CAN3/FD3_C100_0_0x1802F3EF/V2BLifeSig ==
  V2BLifeSig : Inport
  Data Type Conversion : DataTypeConversion  OutDataTypeStr=uint8  RndMeth=Round
  CAN3_V2BLifeSig : Outport
  wires:
  Data Type Conversion/1 -> CAN3_V2BLifeSig/1
  V2BLifeSig/1 -> Data Type Conversion/1

== system halout/HAL_OUT/CAN3/FD3_C100_0_0x1802F3EF/V2BMainPosRlyFlt ==
  V2BMainPosRlyFlt : Inport
  Data Type Conversion : DataTypeConversion  OutDataTypeStr=uint8  RndMeth=Round
  CAN3_V2BMainPosRlyFlt : Outport
  wires:
  Data Type Conversion/1 -> CAN3_V2BMainPosRlyFlt/1
  V2BMainPosRlyFlt/1 -> Data Type Conversion/1

== system halout/HAL_OUT/CAN3/FD3_C100_0_0x1802F3EF/V2BMainPosRlySta ==
  V2BMainPosRlySta : Inport
  Data Type Conversion : DataTypeConversion  OutDataTypeStr=uint8  RndMeth=Round
  CAN3_V2BMainPosRlySta : Outport
  wires:
  Data Type Conversion/1 -> CAN3_V2BMainPosRlySta/1
  V2BMainPosRlySta/1 -> Data Type Conversion/1

== system halout/HAL_OUT/CAN3/FD3_C100_0_0x1802F3EF/V2BOilPosRlyFlt ==
  V2BOilPosRlyFlt : Inport
  Data Type Conversion : DataTypeConversion  OutDataTypeStr=uint8  RndMeth=Round
  CAN3_V2BOilPosRlyFlt : Outport
  wires:
  Data Type Conversion/1 -> CAN3_V2BOilPosRlyFlt/1
  V2BOilPosRlyFlt/1 -> Data Type Conversion/1

== system halout/HAL_OUT/CAN3/FD3_C100_0_0x1802F3EF/V2BOilPosRlySta ==
  V2BOilPosRlySta : Inport
  Data Type Conversion : DataTypeConversion  OutDataTypeStr=uint8  RndMeth=Round
  CAN3_V2BOilPosRlySta : Outport
  wires:
  Data Type Conversion/1 -> CAN3_V2BOilPosRlySta/1
  V2BOilPosRlySta/1 -> Data Type Conversion/1

== system halout/HAL_OUT/CAN3/FD3_C100_0_0x1802F3EF/V2BVehSpd ==
  V2BVehSpd : Inport
  Data Type Conversion : DataTypeConversion  OutDataTypeStr=uint8  RndMeth=Round
  CAN3_V2BVehSpd : Outport
  wires:
  Data Type Conversion/1 -> CAN3_V2BVehSpd/1
  V2BVehSpd/1 -> Data Type Conversion/1

== system halout/HAL_OUT/CAN3/FD3_C10_0_0xCF101D0/DCDCRlyEn ==
  DCDCRlyEn : Inport
  Data Type Conversion : DataTypeConversion  OutDataTypeStr=uint8  RndMeth=Round
  CAN3_DCDCRlyEn : Outport
  wires:
  Data Type Conversion/1 -> CAN3_DCDCRlyEn/1
  DCDCRlyEn/1 -> Data Type Conversion/1

== system halout/HAL_OUT/CAN3/FD3_C10_0_0xCF101D0/EACRlyEn ==
  EACRlyEn : Inport
  Data Type Conversion : DataTypeConversion  OutDataTypeStr=uint8  RndMeth=Round
  CAN3_EACRlyEn : Outport
  wires:
  Data Type Conversion/1 -> CAN3_EACRlyEn/1
  EACRlyEn/1 -> Data Type Conversion/1

== system halout/HAL_OUT/CAN3/FD3_C10_0_0xCF101D0/EHPSRlyEn ==
  EHPSRlyEn : Inport
  Data Type Conversion : DataTypeConversion  OutDataTypeStr=uint8  RndMeth=Round
  CAN3_EHPSRlyEn : Outport
  wires:
  Data Type Conversion/1 -> CAN3_EHPSRlyEn/1
  EHPSRlyEn/1 -> Data Type Conversion/1

== system halout/HAL_OUT/CAN3/FD3_C10_0_0xCF101D0/MCUHVPwrOnOffReq ==
  MCUHVPwrOnOffReq : Inport
  Data Type Conversion : DataTypeConversion  OutDataTypeStr=uint8  RndMeth=Round
  CAN3_MCUHVPwrOnOffReq : Outport
  wires:
  Data Type Conversion/1 -> CAN3_MCUHVPwrOnOffReq/1
  MCUHVPwrOnOffReq/1 -> Data Type Conversion/1

== system halout/HAL_OUT/CAN3/FD3_C10_0_0xCF101D0/VCULife1 ==
  VCULife1 : Inport
  Data Type Conversion : DataTypeConversion  OutDataTypeStr=uint8  RndMeth=Round
  CAN3_VCULife1 : Outport
  wires:
  Data Type Conversion/1 -> CAN3_VCULife1/1
  VCULife1/1 -> Data Type Conversion/1

== system halout/HAL_OUT/CAN3/FD3_C10_1_0xCFF05EF/Byte_0 ==
  VCUMCUCtrlMd : Inport
  VCUMCUEn : Inport  Port=2
  VCUMCUFailRst : Inport  Port=3
  VCUMCUFootBrk : Inport  Port=4
  VCUMCUGearSta : Inport  Port=5
  VCUMCUHandBrk : Inport  Port=6
  BitwiseOR : simulink/Logic and Bit Operations/Bitwise Operator  logicop=OR  UseBitMask=off  NumInputPorts=6  BitMask=bin2dec('11011001')  BitMaskRealWorld=Stored Integer
  SignalPack : FVT_lib/hal/SignalPack  RightShiftCnt=0  BitMask=2^2-1  LeftShiftCnt=2
  SignalPack1 : FVT_lib/hal/SignalPack  RightShiftCnt=0  BitMask=2^1-1  LeftShiftCnt=0
  SignalPack2 : FVT_lib/hal/SignalPack  RightShiftCnt=0  BitMask=2^1-1  LeftShiftCnt=1
  SignalPack3 : FVT_lib/hal/SignalPack  RightShiftCnt=0  BitMask=2^1-1  LeftShiftCnt=6
  SignalPack4 : FVT_lib/hal/SignalPack  RightShiftCnt=0  BitMask=2^2-1  LeftShiftCnt=4
  SignalPack5 : FVT_lib/hal/SignalPack  RightShiftCnt=0  BitMask=2^1-1  LeftShiftCnt=7
  UnitConverter{,1..11} (12 alike) : DataTypeConversion  OutDataTypeStr=uint8  RndMeth=Round
  Byte_0 : Outport
  wires:
  BitwiseOR/1 -> Byte_0/1
  UnitConverter/1 -> BitwiseOR/1
  SignalPack/1 -> UnitConverter/1
  UnitConverter1/1 -> SignalPack/1
  VCUMCUCtrlMd/1 -> UnitConverter1/1
  UnitConverter2/1 -> BitwiseOR/2
  SignalPack1/1 -> UnitConverter2/1
  UnitConverter3/1 -> SignalPack1/1
  VCUMCUEn/1 -> UnitConverter3/1
  UnitConverter4/1 -> BitwiseOR/3
  SignalPack2/1 -> UnitConverter4/1
  UnitConverter5/1 -> SignalPack2/1
  VCUMCUFailRst/1 -> UnitConverter5/1
  UnitConverter6/1 -> BitwiseOR/4
  SignalPack3/1 -> UnitConverter6/1
  UnitConverter7/1 -> SignalPack3/1
  VCUMCUFootBrk/1 -> UnitConverter7/1
  UnitConverter8/1 -> BitwiseOR/5
  SignalPack4/1 -> UnitConverter8/1
  UnitConverter9/1 -> SignalPack4/1
  VCUMCUGearSta/1 -> UnitConverter9/1
  UnitConverter10/1 -> BitwiseOR/6
  SignalPack5/1 -> UnitConverter10/1
  UnitConverter11/1 -> SignalPack5/1
  VCUMCUHandBrk/1 -> UnitConverter11/1

== system halout/HAL_OUT/CAN3/FD3_C10_1_0xCFF05EF/CRC_TX ==
  Byte0 : Inport
  Byte1 : Inport  Port=2
  Byte3 : Inport  Port=3
  Byte4 : Inport  Port=4
  Byte5 : Inport  Port=5
  Byte6 : Inport  Port=6
  Byte7 : Inport  Port=7
  MsgIDLowByte : Inport  Port=8
  MsgIDMidLowByte : Inport  Port=9
  MsgIDMidHighByte : Inport  Port=10
  MsgIDHighByte : Inport  Port=11
  Checksum_J1939_SPN4207 : Stateflow chart  TreatAsAtomicUnit=on
  Rolling_Counter : Stateflow chart  TreatAsAtomicUnit=on
  MsgCntLocal : Outport
  MsgChecksumLocal : Outport  Port=2
  wires:
  MsgIDMidHighByte/1 -> Checksum_J1939_SPN4207/11(MsgIDMidHighByte)
  Byte6/1 -> Checksum_J1939_SPN4207/6(Byte6)
  Byte4/1 -> Checksum_J1939_SPN4207/4(Byte4)
  Checksum_J1939_SPN4207/1(MsgChecksumLocal) -> MsgChecksumLocal/1
  Byte7/1 -> Checksum_J1939_SPN4207/7(Byte7)
  [MsgCntLocal] -> Checksum_J1939_SPN4207/8(MsgCntLocal)
  MsgIDMidLowByte/1 -> Checksum_J1939_SPN4207/10(MsgIDMidLowByte)
  Byte5/1 -> Checksum_J1939_SPN4207/5(Byte5)
  MsgIDLowByte/1 -> Checksum_J1939_SPN4207/9(MsgIDLowByte)
  Byte0/1 -> Checksum_J1939_SPN4207/1(Byte1)
  Byte1/1 -> Checksum_J1939_SPN4207/2(Byte2)
  Byte3/1 -> Checksum_J1939_SPN4207/3(Byte3)
  MsgIDHighByte/1 -> Checksum_J1939_SPN4207/12(MsgIDHighByte)
  Rolling_Counter/1(MsgCntLocal) -> [MsgCntLocal], MsgCntLocal/1

== system halout/HAL_OUT/CAN3/FD3_C10_1_0xCFF05EF/VCUMCUCtrlMd ==
  VCUMCUCtrlMd : Inport
  Data Type Conversion : DataTypeConversion  OutDataTypeStr=uint8  RndMeth=Round
  CAN3_VCUMCUCtrlMd : Outport
  wires:
  Data Type Conversion/1 -> CAN3_VCUMCUCtrlMd/1
  VCUMCUCtrlMd/1 -> Data Type Conversion/1

== system halout/HAL_OUT/CAN3/FD3_C10_1_0xCFF05EF/VCUMCUDemCS ==
  VCUMCUDemCS : Inport
  Data Type Conversion : DataTypeConversion  OutDataTypeStr=uint8  RndMeth=Round
  CAN3_VCUMCUDemCS : Outport
  wires:
  Data Type Conversion/1 -> CAN3_VCUMCUDemCS/1
  VCUMCUDemCS/1 -> Data Type Conversion/1

== system halout/HAL_OUT/CAN3/FD3_C10_1_0xCFF05EF/VCUMCUDemHiPosVal ==
  VCUMCUDemHiPosVal : Inport
  Data Type Conversion : DataTypeConversion  OutDataTypeStr=uint8  RndMeth=Round
  convert_out : FVT_lib/hal/convert_out  gain=40  offset=0
  CAN3_VCUMCUDemHiPosVal : Outport
  wires:
  Data Type Conversion/1 -> CAN3_VCUMCUDemHiPosVal/1
  convert_out/1 -> Data Type Conversion/1
  VCUMCUDemHiPosVal/1 -> convert_out/1

== system halout/HAL_OUT/CAN3/FD3_C10_1_0xCFF05EF/VCUMCUDemLoNegVal ==
  VCUMCUDemLoNegVal : Inport
  Data Type Conversion : DataTypeConversion  OutDataTypeStr=uint8  RndMeth=Round
  convert_out : FVT_lib/hal/convert_out  gain=40  offset=0
  CAN3_VCUMCUDemLoNegVal : Outport
  wires:
  Data Type Conversion/1 -> CAN3_VCUMCUDemLoNegVal/1
  convert_out/1 -> Data Type Conversion/1
  VCUMCUDemLoNegVal/1 -> convert_out/1

== system halout/HAL_OUT/CAN3/FD3_C10_1_0xCFF05EF/VCUMCUDemRC ==
  VCUMCUDemRC : Inport
  Data Type Conversion : DataTypeConversion  OutDataTypeStr=uint8  RndMeth=Round
  CAN3_VCUMCUDemRC : Outport
  wires:
  Data Type Conversion/1 -> CAN3_VCUMCUDemRC/1
  VCUMCUDemRC/1 -> Data Type Conversion/1

== system halout/HAL_OUT/CAN3/FD3_C10_1_0xCFF05EF/VCUMCUDemSpd ==
  VCUMCUDemSpd : Inport
  Data Type Conversion : DataTypeConversion  OutDataTypeStr=uint16  RndMeth=Round
  convert_out : FVT_lib/hal/convert_out  gain=1  offset=-15000
  CAN3_VCUMCUDemSpd : Outport
  wires:
  Data Type Conversion/1 -> CAN3_VCUMCUDemSpd/1
  convert_out/1 -> Data Type Conversion/1
  VCUMCUDemSpd/1 -> convert_out/1

== system halout/HAL_OUT/CAN3/FD3_C10_1_0xCFF05EF/VCUMCUDemTrq ==
  VCUMCUDemTrq : Inport
  Data Type Conversion : DataTypeConversion  OutDataTypeStr=uint16  RndMeth=Round
  convert_out : FVT_lib/hal/convert_out  gain=1  offset=-5000
  CAN3_VCUMCUDemTrq : Outport
  wires:
  Data Type Conversion/1 -> CAN3_VCUMCUDemTrq/1
  convert_out/1 -> Data Type Conversion/1
  VCUMCUDemTrq/1 -> convert_out/1

== system halout/HAL_OUT/CAN3/FD3_C10_1_0xCFF05EF/VCUMCUEn ==
  VCUMCUEn : Inport
  Data Type Conversion : DataTypeConversion  OutDataTypeStr=uint8  RndMeth=Round
  CAN3_VCUMCUEn : Outport
  wires:
  Data Type Conversion/1 -> CAN3_VCUMCUEn/1
  VCUMCUEn/1 -> Data Type Conversion/1

== system halout/HAL_OUT/CAN3/FD3_C10_1_0xCFF05EF/VCUMCUFailRst ==
  VCUMCUFailRst : Inport
  Data Type Conversion : DataTypeConversion  OutDataTypeStr=uint8  RndMeth=Round
  CAN3_VCUMCUFailRst : Outport
  wires:
  Data Type Conversion/1 -> CAN3_VCUMCUFailRst/1
  VCUMCUFailRst/1 -> Data Type Conversion/1

== system halout/HAL_OUT/CAN3/FD3_C10_1_0xCFF05EF/VCUMCUFootBrk ==
  VCUMCUFootBrk : Inport
  Data Type Conversion : DataTypeConversion  OutDataTypeStr=uint8  RndMeth=Round
  CAN3_VCUMCUFootBrk : Outport
  wires:
  Data Type Conversion/1 -> CAN3_VCUMCUFootBrk/1
  VCUMCUFootBrk/1 -> Data Type Conversion/1

== system halout/HAL_OUT/CAN3/FD3_C10_1_0xCFF05EF/VCUMCUGearSta ==
  VCUMCUGearSta : Inport
  Data Type Conversion : DataTypeConversion  OutDataTypeStr=uint8  RndMeth=Round
  CAN3_VCUMCUGearSta : Outport
  wires:
  Data Type Conversion/1 -> CAN3_VCUMCUGearSta/1
  VCUMCUGearSta/1 -> Data Type Conversion/1

== system halout/HAL_OUT/CAN3/FD3_C10_1_0xCFF05EF/VCUMCUHandBrk ==
  VCUMCUHandBrk : Inport
  Data Type Conversion : DataTypeConversion  OutDataTypeStr=uint8  RndMeth=Round
  CAN3_VCUMCUHandBrk : Outport
  wires:
  Data Type Conversion/1 -> CAN3_VCUMCUHandBrk/1
  VCUMCUHandBrk/1 -> Data Type Conversion/1

== system halout/HAL_OUT/CAN3/FD3_C200_0_0x18F003EF/ChrgFault ==
  ChrgFault : Inport
  Data Type Conversion : DataTypeConversion  OutDataTypeStr=uint8  RndMeth=Round
  CAN3_ChrgFault : Outport
  wires:
  Data Type Conversion/1 -> CAN3_ChrgFault/1
  ChrgFault/1 -> Data Type Conversion/1

== system halout/HAL_OUT/CAN3/FD3_C200_0_0x18F003EF/ChrgState ==
  ChrgState : Inport
  Data Type Conversion : DataTypeConversion  OutDataTypeStr=uint8  RndMeth=Round
  CAN3_ChrgState : Outport
  wires:
  Data Type Conversion/1 -> CAN3_ChrgState/1
  ChrgState/1 -> Data Type Conversion/1

== system halout/HAL_OUT/CAN3/FD3_C200_0_0x18F003EF/PowerDownFault ==
  PowerDownFault : Inport
  Data Type Conversion : DataTypeConversion  OutDataTypeStr=uint8  RndMeth=Round
  CAN3_PowerDownFault : Outport
  wires:
  Data Type Conversion/1 -> CAN3_PowerDownFault/1
  PowerDownFault/1 -> Data Type Conversion/1

== system halout/HAL_OUT/CAN3/FD3_C200_0_0x18F003EF/PowerDownState ==
  PowerDownState : Inport
  Data Type Conversion : DataTypeConversion  OutDataTypeStr=uint8  RndMeth=Round
  CAN3_PowerDownState : Outport
  wires:
  Data Type Conversion/1 -> CAN3_PowerDownState/1
  PowerDownState/1 -> Data Type Conversion/1

== system halout/HAL_OUT/CAN3/FD3_C200_0_0x18F003EF/PowerUpFault ==
  PowerUpFault : Inport
  Data Type Conversion : DataTypeConversion  OutDataTypeStr=uint8  RndMeth=Round
  CAN3_PowerUpFault : Outport
  wires:
  Data Type Conversion/1 -> CAN3_PowerUpFault/1
  PowerUpFault/1 -> Data Type Conversion/1

== system halout/HAL_OUT/CAN3/FD3_C200_0_0x18F003EF/PowerUpState ==
  PowerUpState : Inport
  Data Type Conversion : DataTypeConversion  OutDataTypeStr=uint8  RndMeth=Round
  CAN3_PowerUpState : Outport
  wires:
  Data Type Conversion/1 -> CAN3_PowerUpState/1
  PowerUpState/1 -> Data Type Conversion/1

== system halout/HAL_OUT/CAN3/FD3_C200_0_0x18F003EF/SysPowerMode ==
  SysPowerMode : Inport
  Data Type Conversion : DataTypeConversion  OutDataTypeStr=uint8  RndMeth=Round
  CAN3_SysPowerMode : Outport
  wires:
  Data Type Conversion/1 -> CAN3_SysPowerMode/1
  SysPowerMode/1 -> Data Type Conversion/1

== system halout/HAL_OUT/CAN3/FD3_C200_0_0x18F003EF/VCUIGNSta ==
  VCUIGNSta : Inport
  Data Type Conversion : DataTypeConversion  OutDataTypeStr=uint8  RndMeth=Round
  CAN3_VCUIGNSta : Outport
  wires:
  Data Type Conversion/1 -> CAN3_VCUIGNSta/1
  VCUIGNSta/1 -> Data Type Conversion/1

== system halout/HAL_OUT/CAN3/FD3_C200_0_0x18F003EF/VCUIRCSta ==
  VCUIRCSta : Inport
  Data Type Conversion : DataTypeConversion  OutDataTypeStr=uint8  RndMeth=Round
  CAN3_VCUIRCSta : Outport
  wires:
  Data Type Conversion/1 -> CAN3_VCUIRCSta/1
  VCUIRCSta/1 -> Data Type Conversion/1

== system halout/HAL_OUT/CAN3/FD3_C200_0_0x18F003EF/VCUPSSSta ==
  VCUPSSSta : Inport
  Data Type Conversion : DataTypeConversion  OutDataTypeStr=uint8  RndMeth=Round
  CAN3_VCUPSSSta : Outport
  wires:
  Data Type Conversion/1 -> CAN3_VCUPSSSta/1
  VCUPSSSta/1 -> Data Type Conversion/1

== system halout/HAL_OUT/CAN3/FD3_C200_1_0x18F001EF/FDCTHCMEWPPEReqCmd ==
  FDCTHCMEWPPEReqCmd : Inport
  Data Type Conversion : DataTypeConversion  OutDataTypeStr=uint8  RndMeth=Round
  convert_out : FVT_lib/hal/convert_out  gain=25  offset=0
  CAN3_FDC_THCM_EWPPEReq_Cmd : Outport
  wires:
  Data Type Conversion/1 -> CAN3_FDC_THCM_EWPPEReq_Cmd/1
  convert_out/1 -> Data Type Conversion/1
  FDCTHCMEWPPEReqCmd/1 -> convert_out/1

== system halout/HAL_OUT/CAN4/FD4_C100_0_0xCF103D0/DCDCEnDemand ==
  DCDCEnDemand : Inport
  Data Type Conversion : DataTypeConversion  OutDataTypeStr=uint8  RndMeth=Round
  CAN4_DCDCEnDemand : Outport
  wires:
  Data Type Conversion/1 -> CAN4_DCDCEnDemand/1
  DCDCEnDemand/1 -> Data Type Conversion/1

== system halout/HAL_OUT/CAN4/FD4_C100_0_0xCF103D0/EACSpdDemand ==
  EACSpdDemand : Inport
  Data Type Conversion : DataTypeConversion  OutDataTypeStr=uint16  RndMeth=Round
  convert_out : FVT_lib/hal/convert_out  gain=0.5  offset=-5000
  CAN4_EACSpdDemand : Outport
  wires:
  Data Type Conversion/1 -> CAN4_EACSpdDemand/1
  convert_out/1 -> Data Type Conversion/1
  EACSpdDemand/1 -> convert_out/1

== system halout/HAL_OUT/CAN4/FD4_C100_0_0xCF103D0/FDCCHAEACEnDemandCmd ==
  FDCCHAEACEnDemandCmd : Inport
  Data Type Conversion : DataTypeConversion  OutDataTypeStr=uint8  RndMeth=Round
  CAN4_FDC_CHA_EACEnDemand_Cmd : Outport
  wires:
  Data Type Conversion/1 -> CAN4_FDC_CHA_EACEnDemand_Cmd/1
  FDCCHAEACEnDemandCmd/1 -> Data Type Conversion/1

== system halout/HAL_OUT/CAN4/FD4_C100_0_0xCF103D0/FDCEHPSEnDemandCmd ==
  FDCEHPSEnDemandCmd : Inport
  Data Type Conversion : DataTypeConversion  OutDataTypeStr=uint8  RndMeth=Round
  CAN4_FDC_EHPS_EnDemand_Cmd : Outport
  wires:
  Data Type Conversion/1 -> CAN4_FDC_EHPS_EnDemand_Cmd/1
  FDCEHPSEnDemandCmd/1 -> Data Type Conversion/1

== system halout/HAL_OUT/CAN4/FD4_C100_0_0xCF103D0/FDCEHPSSpdDemandCmd ==
  FDCEHPSSpdDemandCmd : Inport
  Data Type Conversion : DataTypeConversion  OutDataTypeStr=uint16  RndMeth=Round
  convert_out : FVT_lib/hal/convert_out  gain=0.5  offset=-5000
  CAN4_FDC_EHPS_SpdDemand_Cmd : Outport
  wires:
  Data Type Conversion/1 -> CAN4_FDC_EHPS_SpdDemand_Cmd/1
  convert_out/1 -> Data Type Conversion/1
  FDCEHPSSpdDemandCmd/1 -> convert_out/1

== system halout/HAL_OUT/CAN4/FD4_C100_0_0xCF103D0/VCULife2 ==
  VCULife2 : Inport
  Data Type Conversion : DataTypeConversion  OutDataTypeStr=uint8  RndMeth=Round
  CAN4_VCULife2 : Outport
  wires:
  Data Type Conversion/1 -> CAN4_VCULife2/1
  VCULife2/1 -> Data Type Conversion/1

== system halout/HAL_OUT/CAN4/FD4_C10_0_0xCF101D0/ACHVPwrOnOffReq ==
  ACHVPwrOnOffReq : Inport
  Data Type Conversion : DataTypeConversion  OutDataTypeStr=uint8  RndMeth=Round
  CAN4_ACHVPwrOnOffReq : Outport
  wires:
  Data Type Conversion/1 -> CAN4_ACHVPwrOnOffReq/1
  ACHVPwrOnOffReq/1 -> Data Type Conversion/1

== system halout/HAL_OUT/CAN4/FD4_C10_0_0xCF101D0/MCUHVPwrOnOffReq ==
  MCUHVPwrOnOffReq : Inport
  Data Type Conversion : DataTypeConversion  OutDataTypeStr=uint8  RndMeth=Round
  CAN4_MCUHVPwrOnOffReq : Outport
  wires:
  Data Type Conversion/1 -> CAN4_MCUHVPwrOnOffReq/1
  MCUHVPwrOnOffReq/1 -> Data Type Conversion/1

== system halout/HAL_OUT/CAN4/FD4_C10_0_0xCF101D0/VCUDCDCEACEHPSRlyEncmd ==
  VCUDCDCEACEHPSRlyEncmd : Inport
  Data Type Conversion : DataTypeConversion  OutDataTypeStr=uint8  RndMeth=Round
  CAN4_VCU_DCDCEACEHPSRlyEn_cmd : Outport
  wires:
  Data Type Conversion/1 -> CAN4_VCU_DCDCEACEHPSRlyEn_cmd/1
  VCUDCDCEACEHPSRlyEncmd/1 -> Data Type Conversion/1

== system halout/HAL_OUT/CAN4/FD4_C10_0_0xCF101D0/VCUDeFogTMSRlyEncmd ==
  VCUDeFogTMSRlyEncmd : Inport
  Data Type Conversion : DataTypeConversion  OutDataTypeStr=uint8  RndMeth=Round
  CAN4_VCU_DeFogTMSRlyEn_cmd : Outport
  wires:
  Data Type Conversion/1 -> CAN4_VCU_DeFogTMSRlyEn_cmd/1
  VCUDeFogTMSRlyEncmd/1 -> Data Type Conversion/1

== system halout/HAL_OUT/CAN4/FD4_C10_0_0xCF101D0/VCULife1 ==
  VCULife1 : Inport
  Data Type Conversion : DataTypeConversion  OutDataTypeStr=uint8  RndMeth=Round
  CAN4_VCULife1 : Outport
  wires:
  Data Type Conversion/1 -> CAN4_VCULife1/1
  VCULife1/1 -> Data Type Conversion/1

== system halout/HAL_OUT/CAN4/FD4_C200_0_0x18F003EF/SysPowerMode ==
  SysPowerMode : Inport
  Data Type Conversion : DataTypeConversion  OutDataTypeStr=uint8  RndMeth=Round
  CAN4_SysPowerMode : Outport
  wires:
  Data Type Conversion/1 -> CAN4_SysPowerMode/1
  SysPowerMode/1 -> Data Type Conversion/1

== system halout/HAL_OUT/CAN4/FD4_C200_0_0x18F003EF/VCUIGNSta ==
  VCUIGNSta : Inport
  Data Type Conversion : DataTypeConversion  OutDataTypeStr=uint8  RndMeth=Round
  CAN4_VCUIGNSta : Outport
  wires:
  Data Type Conversion/1 -> CAN4_VCUIGNSta/1
  VCUIGNSta/1 -> Data Type Conversion/1

== system halout/HAL_OUT/CAN4/FD4_C200_0_0x18F003EF/VCUIRCSta ==
  VCUIRCSta : Inport
  Data Type Conversion : DataTypeConversion  OutDataTypeStr=uint8  RndMeth=Round
  CAN4_VCUIRCSta : Outport
  wires:
  Data Type Conversion/1 -> CAN4_VCUIRCSta/1
  VCUIRCSta/1 -> Data Type Conversion/1

== system halout/HAL_OUT/CAN4/FD4_CE100_0_0x209/FDCBCMBSDBuzzerCmd ==
  FDCBCMBSDBuzzerCmd : Inport
  Data Type Conversion : DataTypeConversion  OutDataTypeStr=uint8  RndMeth=Round
  CAN4_FDC_BCM_BSD_Buzzer_Cmd : Outport
  wires:
  Data Type Conversion/1 -> CAN4_FDC_BCM_BSD_Buzzer_Cmd/1
  FDCBCMBSDBuzzerCmd/1 -> Data Type Conversion/1

== system halout/HAL_OUT/CAN4/FD4_CE100_0_0x209/FDCBCMBrakeCmd ==
  FDCBCMBrakeCmd : Inport
  Data Type Conversion : DataTypeConversion  OutDataTypeStr=uint8  RndMeth=Round
  CAN4_FDC_BCM_Brake_Cmd : Outport
  wires:
  Data Type Conversion/1 -> CAN4_FDC_BCM_Brake_Cmd/1
  FDCBCMBrakeCmd/1 -> Data Type Conversion/1

== system halout/HAL_OUT/CAN4/FD4_CE100_0_0x209/FDCBCMCallBellCmd ==
  FDCBCMCallBellCmd : Inport
  Data Type Conversion : DataTypeConversion  OutDataTypeStr=uint8  RndMeth=Round
  CAN4_FDC_BCM_CallBell_Cmd : Outport
  wires:
  Data Type Conversion/1 -> CAN4_FDC_BCM_CallBell_Cmd/1
  FDCBCMCallBellCmd/1 -> Data Type Conversion/1

== system halout/HAL_OUT/CAN4/FD4_CE100_0_0x209/FDCBCMDVRSignalLCmd ==
  FDCBCMDVRSignalLCmd : Inport
  Data Type Conversion : DataTypeConversion  OutDataTypeStr=uint8  RndMeth=Round
  CAN4_FDC_BCM_DVRSignalL_Cmd : Outport
  wires:
  Data Type Conversion/1 -> CAN4_FDC_BCM_DVRSignalL_Cmd/1
  FDCBCMDVRSignalLCmd/1 -> Data Type Conversion/1

== system halout/HAL_OUT/CAN4/FD4_CE100_0_0x209/FDCBCMDVRSignalRCmd ==
  FDCBCMDVRSignalRCmd : Inport
  Data Type Conversion : DataTypeConversion  OutDataTypeStr=uint8  RndMeth=Round
  CAN4_FDC_BCM_DVRSignalR_Cmd : Outport
  wires:
  Data Type Conversion/1 -> CAN4_FDC_BCM_DVRSignalR_Cmd/1
  FDCBCMDVRSignalRCmd/1 -> Data Type Conversion/1

== system halout/HAL_OUT/CAN4/FD4_CE100_0_0x209/FDCBCMEmExitSWSta ==
  FDCBCMEmExitSWSta : Inport
  Data Type Conversion : DataTypeConversion  OutDataTypeStr=uint8  RndMeth=Round
  CAN4_FDC_BCM_EmExitSW_Sta : Outport
  wires:
  Data Type Conversion/1 -> CAN4_FDC_BCM_EmExitSW_Sta/1
  FDCBCMEmExitSWSta/1 -> Data Type Conversion/1

== system halout/HAL_OUT/CAN4/FD4_CE100_0_0x209/FDCBCMEmSVCmd ==
  FDCBCMEmSVCmd : Inport
  Data Type Conversion : DataTypeConversion  OutDataTypeStr=uint8  RndMeth=Round
  CAN4_FDC_BCM_EmSV_Cmd : Outport
  wires:
  Data Type Conversion/1 -> CAN4_FDC_BCM_EmSV_Cmd/1
  FDCBCMEmSVCmd/1 -> Data Type Conversion/1

== system halout/HAL_OUT/CAN4/FD4_CE100_0_0x209/FDCBCMFDCloseSVCmd ==
  FDCBCMFDCloseSVCmd : Inport
  Data Type Conversion : DataTypeConversion  OutDataTypeStr=uint8  RndMeth=Round
  CAN4_FDC_BCM_FDCloseSV_Cmd : Outport
  wires:
  Data Type Conversion/1 -> CAN4_FDC_BCM_FDCloseSV_Cmd/1
  FDCBCMFDCloseSVCmd/1 -> Data Type Conversion/1

== system halout/HAL_OUT/CAN4/FD4_CE100_0_0x209/FDCBCMFDOpenSVCmd ==
  FDCBCMFDOpenSVCmd : Inport
  Data Type Conversion : DataTypeConversion  OutDataTypeStr=uint8  RndMeth=Round
  CAN4_FDC_BCM_FDOpenSV_Cmd : Outport
  wires:
  Data Type Conversion/1 -> CAN4_FDC_BCM_FDOpenSV_Cmd/1
  FDCBCMFDOpenSVCmd/1 -> Data Type Conversion/1

== system halout/HAL_OUT/CAN4/FD4_CE100_0_0x209/FDCBCMFDoorSta ==
  FDCBCMFDoorSta : Inport
  Data Type Conversion : DataTypeConversion  OutDataTypeStr=uint8  RndMeth=Round
  CAN4_FDC_BCM_FDoor_Sta : Outport
  wires:
  Data Type Conversion/1 -> CAN4_FDC_BCM_FDoor_Sta/1
  FDCBCMFDoorSta/1 -> Data Type Conversion/1

== system halout/HAL_OUT/CAN4/FD4_CE100_0_0x209/FDCBCMHBeamCmd ==
  FDCBCMHBeamCmd : Inport
  Data Type Conversion : DataTypeConversion  OutDataTypeStr=uint8  RndMeth=Round
  CAN4_FDC_BCM_HBeam_Cmd : Outport
  wires:
  Data Type Conversion/1 -> CAN4_FDC_BCM_HBeam_Cmd/1
  FDCBCMHBeamCmd/1 -> Data Type Conversion/1

== system halout/HAL_OUT/CAN4/FD4_CE100_0_0x209/FDCBCMInnerBuzzerCmd ==
  FDCBCMInnerBuzzerCmd : Inport
  Data Type Conversion : DataTypeConversion  OutDataTypeStr=uint8  RndMeth=Round
  CAN4_FDC_BCM_InnerBuzzer_Cmd : Outport
  wires:
  Data Type Conversion/1 -> CAN4_FDC_BCM_InnerBuzzer_Cmd/1
  FDCBCMInnerBuzzerCmd/1 -> Data Type Conversion/1

== system halout/HAL_OUT/CAN4/FD4_CE100_0_0x209/FDCBCMInnerBuzzerModeSta ==
  FDCBCMInnerBuzzerModeSta : Inport
  Data Type Conversion : DataTypeConversion  OutDataTypeStr=uint8  RndMeth=Round
  CAN4_FDC_BCM_InnerBuzzerMode_Sta : Outport
  wires:
  Data Type Conversion/1 -> CAN4_FDC_BCM_InnerBuzzerMode_Sta/1
  FDCBCMInnerBuzzerModeSta/1 -> Data Type Conversion/1

== system halout/HAL_OUT/CAN4/FD4_CE100_0_0x209/FDCBCMInnerCallBellCmd ==
  FDCBCMInnerCallBellCmd : Inport
  Data Type Conversion : DataTypeConversion  OutDataTypeStr=uint8  RndMeth=Round
  CAN4_FDC_BCM_InnerCallBell_Cmd : Outport
  wires:
  Data Type Conversion/1 -> CAN4_FDC_BCM_InnerCallBell_Cmd/1
  FDCBCMInnerCallBellCmd/1 -> Data Type Conversion/1

== system halout/HAL_OUT/CAN4/FD4_CE100_0_0x209/FDCBCMLBSDRCmd ==
  FDCBCMLBSDRCmd : Inport
  Data Type Conversion : DataTypeConversion  OutDataTypeStr=uint8  RndMeth=Round
  CAN4_FDC_BCM_LBSDR_Cmd : Outport
  wires:
  Data Type Conversion/1 -> CAN4_FDC_BCM_LBSDR_Cmd/1
  FDCBCMLBSDRCmd/1 -> Data Type Conversion/1

== system halout/HAL_OUT/CAN4/FD4_CE100_0_0x209/FDCBCMLBSDYCmd ==
  FDCBCMLBSDYCmd : Inport
  Data Type Conversion : DataTypeConversion  OutDataTypeStr=uint8  RndMeth=Round
  CAN4_FDC_BCM_LBSDY_Cmd : Outport
  wires:
  Data Type Conversion/1 -> CAN4_FDC_BCM_LBSDY_Cmd/1
  FDCBCMLBSDYCmd/1 -> Data Type Conversion/1

== system halout/HAL_OUT/CAN4/FD4_CE100_0_0x209/FDCBCMLBeamCmd ==
  FDCBCMLBeamCmd : Inport
  Data Type Conversion : DataTypeConversion  OutDataTypeStr=uint8  RndMeth=Round
  CAN4_FDC_BCM_LBeam_Cmd : Outport
  wires:
  Data Type Conversion/1 -> CAN4_FDC_BCM_LBeam_Cmd/1
  FDCBCMLBeamCmd/1 -> Data Type Conversion/1

== system halout/HAL_OUT/CAN4/FD4_CE100_0_0x209/FDCBCMLDRLCmd ==
  FDCBCMLDRLCmd : Inport
  Data Type Conversion : DataTypeConversion  OutDataTypeStr=uint8  RndMeth=Round
  CAN4_FDC_BCM_LDRL_Cmd : Outport
  wires:
  Data Type Conversion/1 -> CAN4_FDC_BCM_LDRL_Cmd/1
  FDCBCMLDRLCmd/1 -> Data Type Conversion/1

== system halout/HAL_OUT/CAN4/FD4_CE100_0_0x209/FDCBCMLTurnLpCmd ==
  FDCBCMLTurnLpCmd : Inport
  Data Type Conversion : DataTypeConversion  OutDataTypeStr=uint8  RndMeth=Round
  CAN4_FDC_BCM_LTurnLp_Cmd : Outport
  wires:
  Data Type Conversion/1 -> CAN4_FDC_BCM_LTurnLp_Cmd/1
  FDCBCMLTurnLpCmd/1 -> Data Type Conversion/1
